simulink model "ACDCMG_woPV"  (R2022a)
settings: Solver=FixedStepAuto  StartTime=0.0  StopTime=0.2  FixedStep=Ts  MaxStep=1e-2  RelTol=1e-3
InitFcn:
  | Set_parameters_R2018
values from neighbouring files (symbols this model uses):
  D_invs = 0.05    [Set_parameters_R2018.m]
  dis11 = 3    [Set_parameters_R2018.m]
  dis14 = 2    [Set_parameters_R2018.m]
  dis2 = 0.2    [Set_parameters_R2018.m]
  dis3 = 0.15    [Set_parameters_R2018.m]
  dis4 = 0.4    [Set_parameters_R2018.m]
  dis5 = 0.4    [Set_parameters_R2018.m]
  dis6 = 0.4    [Set_parameters_R2018.m]
  dis8 = 2    [Set_parameters_R2018.m]
  Fnom = 60    [Set_parameters_R2018.m]
  H_invs = 6    [Set_parameters_R2018.m]
  max_min = 1    [Set_parameters_R2018.m]
  P_Load_3 = S_Load_3* PF_Load_3    (= 25500)    [Set_parameters_R2018.m]
  P_nom_inv = 3e3    (= 3000)    [Set_parameters_R2018.m]
  Pnom_T1 = 1.5e6    (= 1500000)    [Set_parameters_R2018.m]
  Pnom_T2 = 1.5e6    (= 1500000)    [Set_parameters_R2018.m]
  Pnom_T3 = 4e6    (= 4000000)    [Set_parameters_R2018.m]
  Ql_Load_3 = S_Load_3 * sin(acos(PF_Load_3))    [Set_parameters_R2018.m]
  R_Load_9 = (Vnom_prim * 1.35)^2 / P_Load_9    (= 1084.6153125)    [Set_parameters_R2018.m]
  R_Load_DC = Vnom_DC^2/ P_Load_DC    (= 45)    [Set_parameters_R2018.m]
  Rl = 0.394    [Set_parameters_R2018.m]
  Rls = 0.198    [Set_parameters_R2018.m]
  Ts = Ts_Power    (= 6.94444444444e-06)    [Set_parameters_R2018.m]
  Ts_Control = 6*Ts_Power    (= 4.16666666667e-05)    [Set_parameters_R2018.m]
  Ts_Power = 1/(24*Fnom)/100    (= 6.94444444444e-06)    [Set_parameters_R2018.m]
  V1_LL_T3 = 69e3    (= 69000)    [Set_parameters_R2018.m]
  Vnom_DC = 300    [Set_parameters_R2018.m]
  Vnom_Diesel = 2.4e3    (= 2400)    [Set_parameters_R2018.m]
  Vnom_prim = 13.8e3    (= 13800)    [Set_parameters_R2018.m]
  Vnom_sec = 220    [Set_parameters_R2018.m]
  Vnom_ter_AC_DC = 150    [Set_parameters_R2018.m]
  Xl = 0.1168    [Set_parameters_R2018.m]
  Xls = 0.1089    [Set_parameters_R2018.m]
undefined symbols (not defined in the file or in its folder): D1, Delta, DiscIntNeverNeededParam, ee_sli_rtmsupport, fn, gcbh, Ion, Lithium, S, sigbuilder_block, VnInv
libraries: powerlib_extras x55, spsCurrentMeasurementLib x53, powerlib_meascontrol x42, spsSeriesRLCBranchLib x32, spsVoltageMeasurementLib x31, spsRMSLib x29, spsThreePhaseVIMeasurementLib x24, simulink x21, spsThreePhaseSeriesRLCBranchLib x19, spsPower3phInstantaneousLib x15, spsPowerLib x12, spsGroundLib x11
(part 5 of 9)

== system ACDCMG_woPV/Grid Bi-directional Converter 1.1 300 (DC) // 150 V (AC) P_nom 3kW/Control of Inverter ==
  note: VL-L rms_1
  note: Primary control
  note: Control of Inverter
  Means : Inport
  Bus Selector : BusSelector  OutputSignals=signal1,signal2,signal3,signal4
  Discrete PWM Generator1 : Subsystem  AncestorBlock=|  DialogController=POWERSYS.PowerSysDialog  mask(Discrete PWM Generator){GeneratorMode=3-arm  bridge (6 pulses), Fc=4000, Ts=Ts_Power, Internal=off, mIndex=0.99, Freq=60, Phase=0}
      | powerlib_extras/Discrete 
      | Control Blocks/Discrete
      | PWM Generator
      mask prompts: GeneratorMode "Generator Mode"; Fc "Carrier frequency (Hz):"; Ts "Sample time:"; Internal "Internal generation of modulating signal(s)"; mIndex "Modulation index  (0<m<1) :"; Freq "Frequency of output voltage (Hz)"; Phase "Phase of output voltage (degrees)"
      mask help:
      | This discrete block generates pulses for carrier-based PWM (Pulse Width Modulation), self-commutated IGBTs,GTOs or FETs bridges.
      |
      | Depending on the number of bridge arms selected in the "Generator Mode" parameter, the block can be used either for single-phase or three-phase PWM control.
      mask init:
      | powericon('psbcallbacks',gcb,'Discrete PWM Generator');
      | if Freq==0
      |     Phase=90;
      | end
      | switch GeneratorMode
      | case 1,
      |     Internal_Phase=0;
      |    Signal_PortWidth=1;
      |    Select1_Elements=[1 2];
      |    Select1_PortWidth=2;
      |    Select3_Elements=[1 2];
      |    Select3_PortWidth=4;
      | case 2,
      |     Internal_Phase=0;
      |     Signal_PortWidth=1;
      |     Select1_Elements=[1 2];
      |     Select1_PortWidth=2;
      |     Select3_Elements=[1 2 3 4];
      |     Select3_PortWidth=4;
      | case 3,
      |     Internal_Phase=[0 -2*pi/3 2*pi/3];
      |     Signal_PortWidth=3;
      |     Select1_Elements=[1 4 2 5 3 6];
      |     Select1_PortWidth=6;
      |    Select3_Elements=[1 2 3 4 5 6];
      |    Select3_PortWidth=12;
      | case 4,
      |     Internal_Phase=[0 -2*pi/3 2*pi/3];
      |     Signal_PortWidth=3;
      |     Select1_Elements=[1 4 2 5 3 6];
      |     Select1_PortWidth=6;
      |    Select3_Elements=[1 2 3 4 5 6 7 8 9 10 11 12];
      |    Select3_PortWidth=12;
      | end
      | power_initmask();
      mask Help:
      | The output pulses are a vector (with values=0 or 1). Depending on the selected "Generator Mode", the output vector contains:
      | For a 1-arm  bridge: Two pulses. Pulse 1 is for the upper switch and pulse 2 is for the lower switch.
      | For a 2-arm  bridge: Four pulses. Pulses 1 and 3 are respectively for the upper switches of the first and second arm. Pulses 2 and 4 are for the lower switches.
      | For a 3-arm  bridge: Six pulses. Pulses 1,3 and 5 are respectively for the upper switches of the first,second and third arm. Pulses 2,4 and 6 are for the lower switches.
      | For double 3-arm bridges: Twelve pulses.The first six pulses (pulses 1 to 6) must be sent to the first 3-arm bridge and the last six (pulses 7 to 12) to the second 3-arm bridge.
      | 
      | By selecting "Internal generation" you can can control the modulation index m, frequency and phase of the output voltage  from the internal parameters (m, Freq and Phase). Otherwise, external signals are used for pulse generation. The width of the input vector must be 1 for single phase bridges ( 1-arm or 2-arm)  and 3 for 3-phase bridges  (single or double bridge).
      mask TypeOptions GeneratorMode: 1-arm  bridge (2 pulses) | 2-arm  bridge (4 pulses) | 3-arm  bridge (6 pulses) | Double 3-arm  bridges (12 pulses)
      mask Callback Internal: powericon('psbcallbacks',gcb,'Discrete PWM Generator',[]);
  MI Controller : Subsystem
  Unit Delay4 : UnitDelay  SampleTime=Ts_Power  HasFrameUpgradeWarning=on
  VL-L_1 : Scope  NumInputPorts=2
  Vph_abc : Scope
  Vph_rms_1 : Scope
  u / m : Scope
  Pulses : Outport  VectorParamsAs1DForOutWhenUnconnected=off
  wires:
  MI Controller/2(u / m) -> u / m/1
  Unit Delay4/1 -> Pulses/1
  Discrete PWM Generator1/1(Pulses) -> Unit Delay4/1
  Bus Selector/1 -> Vph_abc/1, MI Controller/1(Vabc)  "<signal1>"
  Bus Selector/2 -> VL-L_1/1  "<signal2>"
  Bus Selector/3 -> VL-L_1/2  "<signal3>"
  Bus Selector/4 -> Vph_rms_1/1  "<signal4>"
  Means/1 -> Bus Selector/1
  MI Controller/1(Vabc_inv) -> Discrete PWM Generator1/1(Uref)

== system ACDCMG_woPV/Grid Bi-directional Converter 1.1 300 (DC) // 150 V (AC) P_nom 3kW1/Control of Inverter ==
  note: VL-L rms_1
  note: Primary control
  note: Control of Inverter
  Means : Inport
  Bus Selector : BusSelector  OutputSignals=signal1,signal2,signal3,signal4
  Discrete PWM Generator1 : Subsystem  AncestorBlock=|  DialogController=POWERSYS.PowerSysDialog  mask(Discrete PWM Generator){GeneratorMode=3-arm  bridge (6 pulses), Fc=4000, Ts=Ts_Power, Internal=off, mIndex=0.99, Freq=60, Phase=0}
      | powerlib_extras/Discrete 
      | Control Blocks/Discrete
      | PWM Generator
      mask prompts: GeneratorMode "Generator Mode"; Fc "Carrier frequency (Hz):"; Ts "Sample time:"; Internal "Internal generation of modulating signal(s)"; mIndex "Modulation index  (0<m<1) :"; Freq "Frequency of output voltage (Hz)"; Phase "Phase of output voltage (degrees)"
      mask help:
      | This discrete block generates pulses for carrier-based PWM (Pulse Width Modulation), self-commutated IGBTs,GTOs or FETs bridges.
      |
      | Depending on the number of bridge arms selected in the "Generator Mode" parameter, the block can be used either for single-phase or three-phase PWM control.
      mask init: same as ACDCMG_woPV/Grid Bi-directional Converter 1.1 300 (DC) // 150 V (AC) P_nom 3kW/Control of Inverter/Discrete PWM Generator1
      mask Help:
      | The output pulses are a vector (with values=0 or 1). Depending on the selected "Generator Mode", the output vector contains:
      | For a 1-arm  bridge: Two pulses. Pulse 1 is for the upper switch and pulse 2 is for the lower switch.
      | For a 2-arm  bridge: Four pulses. Pulses 1 and 3 are respectively for the upper switches of the first and second arm. Pulses 2 and 4 are for the lower switches.
      | For a 3-arm  bridge: Six pulses. Pulses 1,3 and 5 are respectively for the upper switches of the first,second and third arm. Pulses 2,4 and 6 are for the lower switches.
      | For double 3-arm bridges: Twelve pulses.The first six pulses (pulses 1 to 6) must be sent to the first 3-arm bridge and the last six (pulses 7 to 12) to the second 3-arm bridge.
      | 
      | By selecting "Internal generation" you can can control the modulation index m, frequency and phase of the output voltage  from the internal parameters (m, Freq and Phase). Otherwise, external signals are used for pulse generation. The width of the input vector must be 1 for single phase bridges ( 1-arm or 2-arm)  and 3 for 3-phase bridges  (single or double bridge).
      mask TypeOptions GeneratorMode: 1-arm  bridge (2 pulses) | 2-arm  bridge (4 pulses) | 3-arm  bridge (6 pulses) | Double 3-arm  bridges (12 pulses)
      mask Callback Internal: powericon('psbcallbacks',gcb,'Discrete PWM Generator',[]);
  MI Controller : Subsystem
  Unit Delay4 : UnitDelay  SampleTime=Ts_Power  HasFrameUpgradeWarning=on
  VL-L_1 : Scope  NumInputPorts=2
  Vph_abc : Scope
  Vph_rms_1 : Scope
  u / m : Scope
  Pulses : Outport  VectorParamsAs1DForOutWhenUnconnected=off
  wires:
  MI Controller/2(u / m) -> u / m/1
  Unit Delay4/1 -> Pulses/1
  Discrete PWM Generator1/1(Pulses) -> Unit Delay4/1
  Bus Selector/1 -> Vph_abc/1, MI Controller/1(Vabc)  "<signal1>"
  Bus Selector/2 -> VL-L_1/1  "<signal2>"
  Bus Selector/3 -> VL-L_1/2  "<signal3>"
  Bus Selector/4 -> Vph_rms_1/1  "<signal4>"
  Means/1 -> Bus Selector/1
  MI Controller/1(Vabc_inv) -> Discrete PWM Generator1/1(Uref)

== system ACDCMG_woPV/Grid Bi-directional Converter 1.1 300 (DC) // 150 V (AC) P_nom 3kW2/Control of Inverter ==
  note: VL-L rms_1
  note: Primary control
  note: Control of Inverter
  Means : Inport
  Bus Selector : BusSelector  OutputSignals=signal1,signal2,signal3,signal4
  Discrete PWM Generator1 : Subsystem  AncestorBlock=|  DialogController=POWERSYS.PowerSysDialog  mask(Discrete PWM Generator){GeneratorMode=3-arm  bridge (6 pulses), Fc=4000, Ts=Ts_Power, Internal=off, mIndex=0.99, Freq=60, Phase=0}
      | powerlib_extras/Discrete 
      | Control Blocks/Discrete
      | PWM Generator
      mask prompts: GeneratorMode "Generator Mode"; Fc "Carrier frequency (Hz):"; Ts "Sample time:"; Internal "Internal generation of modulating signal(s)"; mIndex "Modulation index  (0<m<1) :"; Freq "Frequency of output voltage (Hz)"; Phase "Phase of output voltage (degrees)"
      mask help:
      | This discrete block generates pulses for carrier-based PWM (Pulse Width Modulation), self-commutated IGBTs,GTOs or FETs bridges.
      |
      | Depending on the number of bridge arms selected in the "Generator Mode" parameter, the block can be used either for single-phase or three-phase PWM control.
      mask init: same as ACDCMG_woPV/Grid Bi-directional Converter 1.1 300 (DC) // 150 V (AC) P_nom 3kW/Control of Inverter/Discrete PWM Generator1
      mask Help:
      | The output pulses are a vector (with values=0 or 1). Depending on the selected "Generator Mode", the output vector contains:
      | For a 1-arm  bridge: Two pulses. Pulse 1 is for the upper switch and pulse 2 is for the lower switch.
      | For a 2-arm  bridge: Four pulses. Pulses 1 and 3 are respectively for the upper switches of the first and second arm. Pulses 2 and 4 are for the lower switches.
      | For a 3-arm  bridge: Six pulses. Pulses 1,3 and 5 are respectively for the upper switches of the first,second and third arm. Pulses 2,4 and 6 are for the lower switches.
      | For double 3-arm bridges: Twelve pulses.The first six pulses (pulses 1 to 6) must be sent to the first 3-arm bridge and the last six (pulses 7 to 12) to the second 3-arm bridge.
      | 
      | By selecting "Internal generation" you can can control the modulation index m, frequency and phase of the output voltage  from the internal parameters (m, Freq and Phase). Otherwise, external signals are used for pulse generation. The width of the input vector must be 1 for single phase bridges ( 1-arm or 2-arm)  and 3 for 3-phase bridges  (single or double bridge).
      mask TypeOptions GeneratorMode: 1-arm  bridge (2 pulses) | 2-arm  bridge (4 pulses) | 3-arm  bridge (6 pulses) | Double 3-arm  bridges (12 pulses)
      mask Callback Internal: powericon('psbcallbacks',gcb,'Discrete PWM Generator',[]);
  MI Controller : Subsystem
  Unit Delay4 : UnitDelay  SampleTime=Ts_Power  HasFrameUpgradeWarning=on
  VL-L_1 : Scope  NumInputPorts=2
  Vph_abc : Scope
  Vph_rms_1 : Scope
  u / m : Scope
  Pulses : Outport  VectorParamsAs1DForOutWhenUnconnected=off
  wires:
  MI Controller/2(u / m) -> u / m/1
  Unit Delay4/1 -> Pulses/1
  Discrete PWM Generator1/1(Pulses) -> Unit Delay4/1
  Bus Selector/1 -> Vph_abc/1, MI Controller/1(Vabc)  "<signal1>"
  Bus Selector/2 -> VL-L_1/1  "<signal2>"
  Bus Selector/3 -> VL-L_1/2  "<signal3>"
  Bus Selector/4 -> Vph_rms_1/1  "<signal4>"
  Means/1 -> Bus Selector/1
  MI Controller/1(Vabc_inv) -> Discrete PWM Generator1/1(Uref)

== system ACDCMG_woPV/Grid Bi-directional Converter 1.2 300 (DC) // 150 V (AC) P_nom 3kW/Control of Inverter ==
  note: VL-L rms_2
  note: Primary control
  note: Control of Inverter
  Bus Selector : BusSelector  Commented=on  OutputSignals=signal1,signal2,signal3,signal4
  Demux3 : Demux  Outputs=3
  Demux4 : Demux  Outputs=3
  Discrete PWM Generator1 : Subsystem  Commented=on  AncestorBlock=|  DialogController=POWERSYS.PowerSysDialog  mask(Discrete PWM Generator){GeneratorMode=3-arm  bridge (6 pulses), Fc=4000, Ts=Ts_Power, Internal=off, mIndex=0.99, Freq=60, Phase=0}
      | powerlib_extras/Discrete 
      | Control Blocks/Discrete
      | PWM Generator
      mask prompts: GeneratorMode "Generator Mode"; Fc "Carrier frequency (Hz):"; Ts "Sample time:"; Internal "Internal generation of modulating signal(s)"; mIndex "Modulation index  (0<m<1) :"; Freq "Frequency of output voltage (Hz)"; Phase "Phase of output voltage (degrees)"
      mask help:
      | This discrete block generates pulses for carrier-based PWM (Pulse Width Modulation), self-commutated IGBTs,GTOs or FETs bridges.
      |
      | Depending on the number of bridge arms selected in the "Generator Mode" parameter, the block can be used either for single-phase or three-phase PWM control.
      mask init: same as ACDCMG_woPV/Grid Bi-directional Converter 1.1 300 (DC) // 150 V (AC) P_nom 3kW/Control of Inverter/Discrete PWM Generator1
      mask Help:
      | The output pulses are a vector (with values=0 or 1). Depending on the selected "Generator Mode", the output vector contains:
      | For a 1-arm  bridge: Two pulses. Pulse 1 is for the upper switch and pulse 2 is for the lower switch.
      | For a 2-arm  bridge: Four pulses. Pulses 1 and 3 are respectively for the upper switches of the first and second arm. Pulses 2 and 4 are for the lower switches.
      | For a 3-arm  bridge: Six pulses. Pulses 1,3 and 5 are respectively for the upper switches of the first,second and third arm. Pulses 2,4 and 6 are for the lower switches.
      | For double 3-arm bridges: Twelve pulses.The first six pulses (pulses 1 to 6) must be sent to the first 3-arm bridge and the last six (pulses 7 to 12) to the second 3-arm bridge.
      | 
      | By selecting "Internal generation" you can can control the modulation index m, frequency and phase of the output voltage  from the internal parameters (m, Freq and Phase). Otherwise, external signals are used for pulse generation. The width of the input vector must be 1 for single phase bridges ( 1-arm or 2-arm)  and 3 for 3-phase bridges  (single or double bridge).
      mask TypeOptions GeneratorMode: 1-arm  bridge (2 pulses) | 2-arm  bridge (4 pulses) | 3-arm  bridge (6 pulses) | Double 3-arm  bridges (12 pulses)
      mask Callback Internal: powericon('psbcallbacks',gcb,'Discrete PWM Generator',[]);
  Goto : Goto  Commented=on  GotoTag=PWM
  MI Controller : Subsystem  Commented=on
  Mux2 : Mux  Inputs=2
  PQ_B1 : Scope
  "P_Q(kW, kvar)1" : Display
      settings: Format=bank  Decimation=2000
  Positive-Sequence Active & Reactive Power1 : Subsystem  AncestorBlock=|  DialogController=POWERSYS.PowerSysDialog  mask(Discrete 3-phase Positive-Sequence Active & Reactive Power){Freq=60, Par_Vinit=[0 0], Par_Iinit=[0 0], Ts=5e-6}
      | powerlib_extras/Discrete
      | Measurements/Discrete 3-phase 
      | Positive-Sequence 
      | Active & Reactive Power
      mask prompts: Freq "Fundamental frequency (Hz):"; Par_Vinit "Voltage initial input: [ Mag  Phase(degrees) ]"; Par_Iinit "Current initial input: [ Mag  Phase(degrees) ]"; Ts "Sample time:"
      mask help:
      | Measure the three-phase active power P and reactive power Q associated with a periodic set of three-phase voltages and currents which may contain harmonics. P and Q are calculated by evaluating the fundamental values (positive-sequence) of the input voltages and currents with a running window over one cycle of the fundamental frequency.
      |
      | Current flowing into an RL circuit will produce  positive active and reactive powers.
      |
      | Vabc input: Three-phase instantaneous voltage (V)
      | Iabc input: Three-phase instantaneous current (A)
      |
      | Output 1: Vector [Mag_V(V) Mag_I(A)] of the fundamental values of the voltage & current (peak values of the positive-sequence)
      | Output 2: 3-phase PQ measurement vector [P(W) Q (var)] evaluated at the fundamental frequency.
      |
      | For the first cycle of simulation, the outputs are held constant using the values specified by the parameters "Initial input".
      mask init:
      | power_initmask();
      mask Help: This block is part of a subset of blocks in the Extras library that does not have documentation associated with it, other than the block mask description.
      mask Display: disp('')
  RMS_VI2 : Scope
  RMS_V_I1 : Display
      settings: Format=bank  Decimation=2000
  Scope1 : Scope  NumInputPorts=2
  Scope2 : Scope
  Scope6 : Scope  NumInputPorts=2
  Terminator{1..6} (6 alike) : Terminator
  Unit Delay4 : UnitDelay  Commented=on  SampleTime=Ts_Power  HasFrameUpgradeWarning=on
  V/F : Subsystem
  VL-L_2 : Scope  Commented=on  NumInputPorts=2
  Vph_rms_2 : Scope  Commented=on
  m2 : Scope  Commented=on
  m_2 : Scope  Commented=on
  Pulses : Outport  VectorParamsAs1DForOutWhenUnconnected=off
  wires:
  MI Controller/2(m) -> m_2/1
  Discrete PWM Generator1/1(Pulses) -> Unit Delay4/1
  MI Controller/1(Vabc_inv) -> Discrete PWM Generator1/1(Uref)
  Bus Selector/1 -> m2/1, MI Controller/1(Vabc)  "<signal1>"
  Bus Selector/2 -> VL-L_2/1  "<signal2>"
  Bus Selector/3 -> VL-L_2/2  "<signal3>"
  Bus Selector/4 -> Vph_rms_2/1  "<signal4>"
  [Udc] -> V/F/4(Udc)
  Demux3/2 -> Terminator1/1
  Demux4/3 -> Terminator6/1
  [i] -> V/F/3(i)
  Demux4/2 -> Terminator5/1
  Demux4/1 -> Mux2/2
  Demux3/3 -> Terminator4/1
  [io] -> Scope1/2, Positive-Sequence Active & Reactive Power1/2(Iabc)
  Mux2/1 -> Scope2/1
  Demux3/1 -> Mux2/1
  Positive-Sequence Active & Reactive Power1/2(P_Q(kW)) -> PQ_B1/1, "P_Q(kW, kvar)1"/1
  Positive-Sequence Active & Reactive Power1/4(PF) -> Terminator3/1
  Positive-Sequence Active & Reactive Power1/3(Phase_V_I) -> Terminator2/1
  Positive-Sequence Active & Reactive Power1/1(RMS_V_I) -> RMS_V_I1/1, RMS_VI2/1
  [e] -> Scope1/1, Positive-Sequence Active & Reactive Power1/1(Vabc)
  [e] -> Scope6/1, Demux3/1, V/F/1(e)
  [io] -> Scope6/2, Demux4/1, V/F/2(io)
  V/F/1(Pulses) -> Pulses/1

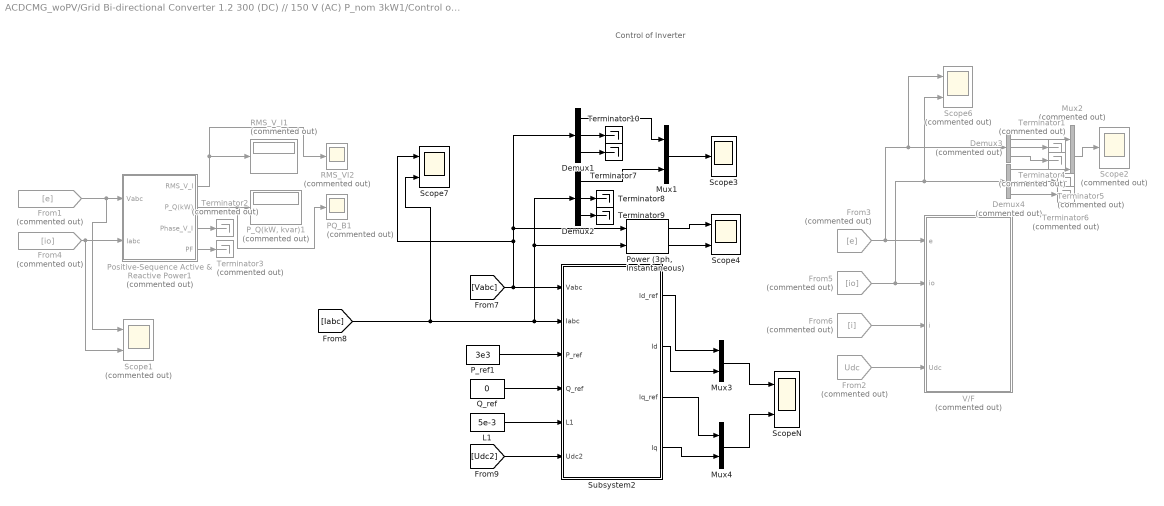
== system ACDCMG_woPV/Grid Bi-directional Converter 1.2 300 (DC) // 150 V (AC) P_nom 3kW1/Control of Inverter ==
  note: Control of Inverter
  Demux1 : Demux  Outputs=3
  Demux2 : Demux  Outputs=3
  Demux3 : Demux  Commented=on  Outputs=3
  Demux4 : Demux  Commented=on  Outputs=3
  From1 : From  Commented=on  GotoTag=e  TagVisibility=global
      settings: CloseFcn=tagdialog Close
  From2 : From  Commented=on  GotoTag=Udc  TagVisibility=global
  From3 : From  Commented=on  GotoTag=e  TagVisibility=global
  From4 : From  Commented=on  GotoTag=io  TagVisibility=global
      settings: CloseFcn=tagdialog Close
  From5 : From  Commented=on  GotoTag=io  TagVisibility=global
  From6 : From  Commented=on  GotoTag=i  TagVisibility=global
  L1 : Constant  Value=5e-3
  Mux1 : Mux  Inputs=2
  Mux2 : Mux  Commented=on  Inputs=2
  Mux3 : Mux  Inputs=2
  Mux4 : Mux  Inputs=2
  PQ_B1 : Scope  Commented=on
  "P_Q(kW, kvar)1" : Display  Commented=on
      settings: Format=bank  Decimation=2000
  P_ref1 : Constant  Value=3e3
  Positive-Sequence Active & Reactive Power1 : Subsystem  Commented=on  AncestorBlock=|  DialogController=POWERSYS.PowerSysDialog  mask(Discrete 3-phase Positive-Sequence Active & Reactive Power){Freq=60, Par_Vinit=[0 0], Par_Iinit=[0 0], Ts=5e-6}
      | powerlib_extras/Discrete
      | Measurements/Discrete 3-phase 
      | Positive-Sequence 
      | Active & Reactive Power
      mask prompts: Freq "Fundamental frequency (Hz):"; Par_Vinit "Voltage initial input: [ Mag  Phase(degrees) ]"; Par_Iinit "Current initial input: [ Mag  Phase(degrees) ]"; Ts "Sample time:"
      mask help:
      | Measure the three-phase active power P and reactive power Q associated with a periodic set of three-phase voltages and currents which may contain harmonics. P and Q are calculated by evaluating the fundamental values (positive-sequence) of the input voltages and currents with a running window over one cycle of the fundamental frequency.
      |
      | Current flowing into an RL circuit will produce  positive active and reactive powers.
      |
      | Vabc input: Three-phase instantaneous voltage (V)
      | Iabc input: Three-phase instantaneous current (A)
      |
      | Output 1: Vector [Mag_V(V) Mag_I(A)] of the fundamental values of the voltage & current (peak values of the positive-sequence)
      | Output 2: 3-phase PQ measurement vector [P(W) Q (var)] evaluated at the fundamental frequency.
      |
      | For the first cycle of simulation, the outputs are held constant using the values specified by the parameters "Initial input".
      mask init:
      | power_initmask();
      mask Help: This block is part of a subset of blocks in the Extras library that does not have documentation associated with it, other than the block mask description.
      mask Display: disp('')
  "Power (3ph, Instantaneous)" : powerlib_meascontrol/Measurements/Power (3ph, Instantaneous)
  Q_ref : Constant  Value=0
  RMS_VI2 : Scope  Commented=on
  RMS_V_I1 : Display  Commented=on
      settings: Format=bank  Decimation=2000
  Scope1 : Scope  Commented=on  NumInputPorts=2
  Scope2 : Scope  Commented=on
  Scope3 : Scope
  Scope4 : Scope  NumInputPorts=2
  Scope6 : Scope  Commented=on  NumInputPorts=2
  Scope7 : Scope  NumInputPorts=2
  ScopeN : Scope  NumInputPorts=2
  Subsystem2 : Subsystem  mask{Kp=21, Ki=101, Kd=0}
      mask prompts: Kp "Proportional gain (Kp):"; Ki "Integral gain (Ki):"; Kd "Derivative gain (Kd):"
  Terminator{1..6} (6 alike) : Terminator  Commented=on
  Terminator{7..10} (4 alike) : Terminator
  V/F : Subsystem  Commented=on
  wires:
  From2/1 -> V/F/4(Udc)
  Demux3/2 -> Terminator1/1
  Demux4/3 -> Terminator6/1
  From6/1 -> V/F/3(i)
  Demux4/2 -> Terminator5/1
  Demux4/1 -> Mux2/2
  Demux3/3 -> Terminator4/1
  From4/1 -> Scope1/2, Positive-Sequence Active & Reactive Power1/2(Iabc)
  Mux2/1 -> Scope2/1
  Demux3/1 -> Mux2/1
  Positive-Sequence Active & Reactive Power1/2(P_Q(kW)) -> PQ_B1/1, "P_Q(kW, kvar)1"/1
  Positive-Sequence Active & Reactive Power1/4(PF) -> Terminator3/1
  Positive-Sequence Active & Reactive Power1/3(Phase_V_I) -> Terminator2/1
  Positive-Sequence Active & Reactive Power1/1(RMS_V_I) -> RMS_V_I1/1, RMS_VI2/1
  From1/1 -> Scope1/1, Positive-Sequence Active & Reactive Power1/1(Vabc)
  From3/1 -> Scope6/1, Demux3/1, V/F/1(e)
  From5/1 -> Scope6/2, Demux4/1, V/F/2(io)
  Q_ref/1 -> Subsystem2/4(Q_ref)
  [Vabc] -> Subsystem2/1(Vabc), Scope7/1, Demux1/1, "Power (3ph, Instantaneous)"/1
  Demux2/3 -> Terminator9/1
  Demux1/2 -> Terminator10/1
  [Udc2] -> Subsystem2/6(Udc2)
  P_ref1/1 -> Subsystem2/3(P_ref)
  Demux2/2 -> Terminator8/1
  "Power (3ph, Instantaneous)"/2 -> Scope4/2
  "Power (3ph, Instantaneous)"/1 -> Scope4/1
  Subsystem2/3(Iq_ref) -> Mux4/1
  Subsystem2/2(Id) -> Mux3/2
  Demux2/1 -> Mux1/2
  Mux1/1 -> Scope3/1
  L1/1 -> Subsystem2/5(L1)
  Mux3/1 -> ScopeN/1
  Subsystem2/4(Iq) -> Mux4/2
  [Iabc] -> Scope7/2, Demux2/1, "Power (3ph, Instantaneous)"/2, Subsystem2/2(Iabc)
  Subsystem2/1(Id_ref) -> Mux3/1
  Mux4/1 -> ScopeN/2
  Demux1/3 -> Terminator7/1
  Demux1/1 -> Mux1/1

== system ACDCMG_woPV/Grid Bi-directional Converter 1.2 300 (DC) // 150 V (AC) P_nom 3kW1/Power Measurement (Three-Phase) ==
  V : Inport
  I : Inport  Port=2
  Continuous : Subsystem  VariantControl=Continuous
  Discrete : Subsystem  VariantControl=Discrete
  P : Outport  VectorParamsAs1DForOutWhenUnconnected=off
  Q : Outport  Port=2  VectorParamsAs1DForOutWhenUnconnected=off

== system ACDCMG_woPV/Grid Bi-directional Converter 1.2 300 (DC) // 150 V (AC) P_nom 3kW2/Control of Inverter ==
  note: VL-L rms_2
  note: Primary control
  note: Control of Inverter
  Bus Selector : BusSelector  Commented=on  OutputSignals=signal1,signal2,signal3,signal4
  Demux3 : Demux  Outputs=3
  Demux4 : Demux  Outputs=3
  Discrete PWM Generator1 : Subsystem  Commented=on  AncestorBlock=|  DialogController=POWERSYS.PowerSysDialog  mask(Discrete PWM Generator){GeneratorMode=3-arm  bridge (6 pulses), Fc=4000, Ts=Ts_Power, Internal=off, mIndex=0.99, Freq=60, Phase=0}
      | powerlib_extras/Discrete 
      | Control Blocks/Discrete
      | PWM Generator
      mask prompts: GeneratorMode "Generator Mode"; Fc "Carrier frequency (Hz):"; Ts "Sample time:"; Internal "Internal generation of modulating signal(s)"; mIndex "Modulation index  (0<m<1) :"; Freq "Frequency of output voltage (Hz)"; Phase "Phase of output voltage (degrees)"
      mask help:
      | This discrete block generates pulses for carrier-based PWM (Pulse Width Modulation), self-commutated IGBTs,GTOs or FETs bridges.
      |
      | Depending on the number of bridge arms selected in the "Generator Mode" parameter, the block can be used either for single-phase or three-phase PWM control.
      mask init: same as ACDCMG_woPV/Grid Bi-directional Converter 1.1 300 (DC) // 150 V (AC) P_nom 3kW/Control of Inverter/Discrete PWM Generator1
      mask Help:
      | The output pulses are a vector (with values=0 or 1). Depending on the selected "Generator Mode", the output vector contains:
      | For a 1-arm  bridge: Two pulses. Pulse 1 is for the upper switch and pulse 2 is for the lower switch.
      | For a 2-arm  bridge: Four pulses. Pulses 1 and 3 are respectively for the upper switches of the first and second arm. Pulses 2 and 4 are for the lower switches.
      | For a 3-arm  bridge: Six pulses. Pulses 1,3 and 5 are respectively for the upper switches of the first,second and third arm. Pulses 2,4 and 6 are for the lower switches.
      | For double 3-arm bridges: Twelve pulses.The first six pulses (pulses 1 to 6) must be sent to the first 3-arm bridge and the last six (pulses 7 to 12) to the second 3-arm bridge.
      | 
      | By selecting "Internal generation" you can can control the modulation index m, frequency and phase of the output voltage  from the internal parameters (m, Freq and Phase). Otherwise, external signals are used for pulse generation. The width of the input vector must be 1 for single phase bridges ( 1-arm or 2-arm)  and 3 for 3-phase bridges  (single or double bridge).
      mask TypeOptions GeneratorMode: 1-arm  bridge (2 pulses) | 2-arm  bridge (4 pulses) | 3-arm  bridge (6 pulses) | Double 3-arm  bridges (12 pulses)
      mask Callback Internal: powericon('psbcallbacks',gcb,'Discrete PWM Generator',[]);
  Goto : Goto  Commented=on  GotoTag=PWM
  MI Controller : Subsystem  Commented=on
  Mux2 : Mux  Inputs=2
  PQ_B1 : Scope
  "P_Q(kW, kvar)1" : Display
      settings: Format=bank  Decimation=2000
  Positive-Sequence Active & Reactive Power1 : Subsystem  AncestorBlock=|  DialogController=POWERSYS.PowerSysDialog  mask(Discrete 3-phase Positive-Sequence Active & Reactive Power){Freq=60, Par_Vinit=[0 0], Par_Iinit=[0 0], Ts=5e-6}
      | powerlib_extras/Discrete
      | Measurements/Discrete 3-phase 
      | Positive-Sequence 
      | Active & Reactive Power
      mask prompts: Freq "Fundamental frequency (Hz):"; Par_Vinit "Voltage initial input: [ Mag  Phase(degrees) ]"; Par_Iinit "Current initial input: [ Mag  Phase(degrees) ]"; Ts "Sample time:"
      mask help:
      | Measure the three-phase active power P and reactive power Q associated with a periodic set of three-phase voltages and currents which may contain harmonics. P and Q are calculated by evaluating the fundamental values (positive-sequence) of the input voltages and currents with a running window over one cycle of the fundamental frequency.
      |
      | Current flowing into an RL circuit will produce  positive active and reactive powers.
      |
      | Vabc input: Three-phase instantaneous voltage (V)
      | Iabc input: Three-phase instantaneous current (A)
      |
      | Output 1: Vector [Mag_V(V) Mag_I(A)] of the fundamental values of the voltage & current (peak values of the positive-sequence)
      | Output 2: 3-phase PQ measurement vector [P(W) Q (var)] evaluated at the fundamental frequency.
      |
      | For the first cycle of simulation, the outputs are held constant using the values specified by the parameters "Initial input".
      mask init:
      | power_initmask();
      mask Help: This block is part of a subset of blocks in the Extras library that does not have documentation associated with it, other than the block mask description.
      mask Display: disp('')
  RMS_VI2 : Scope
  RMS_V_I1 : Display
      settings: Format=bank  Decimation=2000
  Scope1 : Scope  NumInputPorts=2
  Scope2 : Scope
  Scope6 : Scope  NumInputPorts=2
  Terminator{1..6} (6 alike) : Terminator
  Unit Delay4 : UnitDelay  Commented=on  SampleTime=Ts_Power  HasFrameUpgradeWarning=on
  V/F : Subsystem
  VL-L_2 : Scope  Commented=on  NumInputPorts=2
  Vph_rms_2 : Scope  Commented=on
  m2 : Scope  Commented=on
  m_2 : Scope  Commented=on
  Pulses : Outport  VectorParamsAs1DForOutWhenUnconnected=off
  wires:
  MI Controller/2(m) -> m_2/1
  Discrete PWM Generator1/1(Pulses) -> Unit Delay4/1
  MI Controller/1(Vabc_inv) -> Discrete PWM Generator1/1(Uref)
  Bus Selector/1 -> m2/1, MI Controller/1(Vabc)  "<signal1>"
  Bus Selector/2 -> VL-L_2/1  "<signal2>"
  Bus Selector/3 -> VL-L_2/2  "<signal3>"
  Bus Selector/4 -> Vph_rms_2/1  "<signal4>"
  [Udc] -> V/F/4(Udc)
  Demux3/2 -> Terminator1/1
  Demux4/3 -> Terminator6/1
  [i] -> V/F/3(i)
  Demux4/2 -> Terminator5/1
  Demux4/1 -> Mux2/2
  Demux3/3 -> Terminator4/1
  [io] -> Scope1/2, Positive-Sequence Active & Reactive Power1/2(Iabc)
  Mux2/1 -> Scope2/1
  Demux3/1 -> Mux2/1
  Positive-Sequence Active & Reactive Power1/2(P_Q(kW)) -> PQ_B1/1, "P_Q(kW, kvar)1"/1
  Positive-Sequence Active & Reactive Power1/4(PF) -> Terminator3/1
  Positive-Sequence Active & Reactive Power1/3(Phase_V_I) -> Terminator2/1
  Positive-Sequence Active & Reactive Power1/1(RMS_V_I) -> RMS_V_I1/1, RMS_VI2/1
  [e] -> Scope1/1, Positive-Sequence Active & Reactive Power1/1(Vabc)
  [e] -> Scope6/1, Demux3/1, V/F/1(e)
  [io] -> Scope6/2, Demux4/1, V/F/2(io)
  V/F/1(Pulses) -> Pulses/1

== system ACDCMG_woPV/Grid Bi-directional Converter 1.2 300 (DC) // 150 V (AC) P_nom 3kW3/Control of Inverter ==
  note: Control of Inverter
  Demux3 : Demux  Outputs=3
  Demux4 : Demux  Outputs=3
  From1 : From  Commented=on  GotoTag=e  TagVisibility=global
      settings: CloseFcn=tagdialog Close
  From4 : From  Commented=on  GotoTag=io  TagVisibility=global
      settings: CloseFcn=tagdialog Close
  Mux2 : Mux  Inputs=2
  PQ_B1 : Scope  Commented=on
  "P_Q(kW, kvar)1" : Display  Commented=on
      settings: Format=bank  Decimation=2000
  Positive-Sequence Active & Reactive Power1 : Subsystem  Commented=on  AncestorBlock=|  DialogController=POWERSYS.PowerSysDialog  mask(Discrete 3-phase Positive-Sequence Active & Reactive Power){Freq=60, Par_Vinit=[0 0], Par_Iinit=[0 0], Ts=5e-6}
      | powerlib_extras/Discrete
      | Measurements/Discrete 3-phase 
      | Positive-Sequence 
      | Active & Reactive Power
      mask prompts: Freq "Fundamental frequency (Hz):"; Par_Vinit "Voltage initial input: [ Mag  Phase(degrees) ]"; Par_Iinit "Current initial input: [ Mag  Phase(degrees) ]"; Ts "Sample time:"
      mask help:
      | Measure the three-phase active power P and reactive power Q associated with a periodic set of three-phase voltages and currents which may contain harmonics. P and Q are calculated by evaluating the fundamental values (positive-sequence) of the input voltages and currents with a running window over one cycle of the fundamental frequency.
      |
      | Current flowing into an RL circuit will produce  positive active and reactive powers.
      |
      | Vabc input: Three-phase instantaneous voltage (V)
      | Iabc input: Three-phase instantaneous current (A)
      |
      | Output 1: Vector [Mag_V(V) Mag_I(A)] of the fundamental values of the voltage & current (peak values of the positive-sequence)
      | Output 2: 3-phase PQ measurement vector [P(W) Q (var)] evaluated at the fundamental frequency.
      |
      | For the first cycle of simulation, the outputs are held constant using the values specified by the parameters "Initial input".
      mask init:
      | power_initmask();
      mask Help: This block is part of a subset of blocks in the Extras library that does not have documentation associated with it, other than the block mask description.
      mask Display: disp('')
  RMS_VI2 : Scope  Commented=on
  RMS_V_I1 : Display  Commented=on
      settings: Format=bank  Decimation=2000
  Scope1 : Scope  Commented=on  NumInputPorts=2
  Scope2 : Scope
  Scope6 : Scope  NumInputPorts=2
  Terminator{1,4..6} (4 alike) : Terminator
  Terminator2 : Terminator  Commented=on
  Terminator3 : Terminator  Commented=on
  V/F : Subsystem
  wires:
  [Udc] -> V/F/4(Udc)
  Demux3/2 -> Terminator1/1
  Demux4/3 -> Terminator6/1
  [i] -> V/F/3(i)
  Demux4/2 -> Terminator5/1
  Demux4/1 -> Mux2/2
  Demux3/3 -> Terminator4/1
  From4/1 -> Scope1/2, Positive-Sequence Active & Reactive Power1/2(Iabc)
  Mux2/1 -> Scope2/1
  Demux3/1 -> Mux2/1
  Positive-Sequence Active & Reactive Power1/2(P_Q(kW)) -> PQ_B1/1, "P_Q(kW, kvar)1"/1
  Positive-Sequence Active & Reactive Power1/4(PF) -> Terminator3/1
  Positive-Sequence Active & Reactive Power1/3(Phase_V_I) -> Terminator2/1
  Positive-Sequence Active & Reactive Power1/1(RMS_V_I) -> RMS_V_I1/1, RMS_VI2/1
  From1/1 -> Scope1/1, Positive-Sequence Active & Reactive Power1/1(Vabc)
  [e] -> Scope6/1, Demux3/1, V/F/1(e)
  [io] -> Scope6/2, Demux4/1, V/F/2(io)

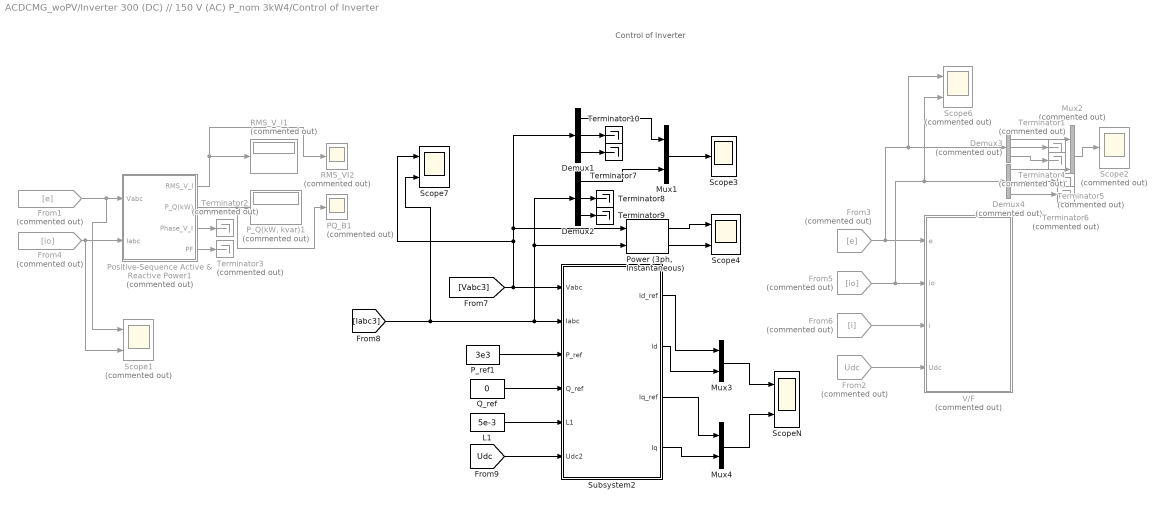
== system ACDCMG_woPV/Inverter 300 (DC) // 150 V (AC) P_nom 3kW4/Control of Inverter ==
  note: Control of Inverter
  Demux1 : Demux  Outputs=3
  Demux2 : Demux  Outputs=3
  Demux3 : Demux  Commented=on  Outputs=3
  Demux4 : Demux  Commented=on  Outputs=3
  From1 : From  Commented=on  GotoTag=e  TagVisibility=global
      settings: CloseFcn=tagdialog Close
  From2 : From  Commented=on  GotoTag=Udc  TagVisibility=global
  From3 : From  Commented=on  GotoTag=e  TagVisibility=global
  From4 : From  Commented=on  GotoTag=io  TagVisibility=global
      settings: CloseFcn=tagdialog Close
  From5 : From  Commented=on  GotoTag=io  TagVisibility=global
  From6 : From  Commented=on  GotoTag=i  TagVisibility=global
  L1 : Constant  Value=5e-3
  Mux1 : Mux  Inputs=2
  Mux2 : Mux  Commented=on  Inputs=2
  Mux3 : Mux  Inputs=2
  Mux4 : Mux  Inputs=2
  PQ_B1 : Scope  Commented=on
  "P_Q(kW, kvar)1" : Display  Commented=on
      settings: Format=bank  Decimation=2000
  P_ref1 : Constant  Value=3e3
  Positive-Sequence Active & Reactive Power1 : Subsystem  Commented=on  AncestorBlock=|  DialogController=POWERSYS.PowerSysDialog  mask(Discrete 3-phase Positive-Sequence Active & Reactive Power){Freq=60, Par_Vinit=[0 0], Par_Iinit=[0 0], Ts=5e-6}
      | powerlib_extras/Discrete
      | Measurements/Discrete 3-phase 
      | Positive-Sequence 
      | Active & Reactive Power
      mask prompts: Freq "Fundamental frequency (Hz):"; Par_Vinit "Voltage initial input: [ Mag  Phase(degrees) ]"; Par_Iinit "Current initial input: [ Mag  Phase(degrees) ]"; Ts "Sample time:"
      mask help:
      | Measure the three-phase active power P and reactive power Q associated with a periodic set of three-phase voltages and currents which may contain harmonics. P and Q are calculated by evaluating the fundamental values (positive-sequence) of the input voltages and currents with a running window over one cycle of the fundamental frequency.
      |
      | Current flowing into an RL circuit will produce  positive active and reactive powers.
      |
      | Vabc input: Three-phase instantaneous voltage (V)
      | Iabc input: Three-phase instantaneous current (A)
      |
      | Output 1: Vector [Mag_V(V) Mag_I(A)] of the fundamental values of the voltage & current (peak values of the positive-sequence)
      | Output 2: 3-phase PQ measurement vector [P(W) Q (var)] evaluated at the fundamental frequency.
      |
      | For the first cycle of simulation, the outputs are held constant using the values specified by the parameters "Initial input".
      mask init:
      | power_initmask();
      mask Help: This block is part of a subset of blocks in the Extras library that does not have documentation associated with it, other than the block mask description.
      mask Display: disp('')
  "Power (3ph, Instantaneous)" : spsPower3phInstantaneousLib/Power (3ph, Instantaneous)
  Q_ref : Constant  Value=0
  RMS_VI2 : Scope  Commented=on
  RMS_V_I1 : Display  Commented=on
      settings: Format=bank  Decimation=2000
  Scope1 : Scope  Commented=on  NumInputPorts=2
  Scope2 : Scope  Commented=on
  Scope3 : Scope
  Scope4 : Scope  NumInputPorts=2
  Scope6 : Scope  Commented=on  NumInputPorts=2
  Scope7 : Scope  NumInputPorts=2
  ScopeN : Scope  NumInputPorts=2
  Subsystem2 : Subsystem  mask{Kp=21, Ki=101, Kd=0}
      mask prompts: Kp "Proportional gain (Kp):"; Ki "Integral gain (Ki):"; Kd "Derivative gain (Kd):"
  Terminator{1..6} (6 alike) : Terminator  Commented=on
  Terminator{7..10} (4 alike) : Terminator
  V/F : Subsystem  Commented=on
  wires:
  From2/1 -> V/F/4(Udc)
  Demux3/2 -> Terminator1/1
  Demux4/3 -> Terminator6/1
  From6/1 -> V/F/3(i)
  Demux4/2 -> Terminator5/1
  Demux4/1 -> Mux2/2
  Demux3/3 -> Terminator4/1
  From4/1 -> Scope1/2, Positive-Sequence Active & Reactive Power1/2(Iabc)
  Mux2/1 -> Scope2/1
  Demux3/1 -> Mux2/1
  Positive-Sequence Active & Reactive Power1/2(P_Q(kW)) -> PQ_B1/1, "P_Q(kW, kvar)1"/1
  Positive-Sequence Active & Reactive Power1/4(PF) -> Terminator3/1
  Positive-Sequence Active & Reactive Power1/3(Phase_V_I) -> Terminator2/1
  Positive-Sequence Active & Reactive Power1/1(RMS_V_I) -> RMS_V_I1/1, RMS_VI2/1
  From1/1 -> Scope1/1, Positive-Sequence Active & Reactive Power1/1(Vabc)
  From3/1 -> Scope6/1, Demux3/1, V/F/1(e)
  From5/1 -> Scope6/2, Demux4/1, V/F/2(io)
  Q_ref/1 -> Subsystem2/4(Q_ref)
  [Vabc3] -> Subsystem2/1(Vabc), Scope7/1, Demux1/1, "Power (3ph, Instantaneous)"/1
  Demux2/3 -> Terminator9/1
  Demux1/2 -> Terminator10/1
  [Udc] -> Subsystem2/6(Udc2)
  P_ref1/1 -> Subsystem2/3(P_ref)
  Demux2/2 -> Terminator8/1
  "Power (3ph, Instantaneous)"/2 -> Scope4/2
  "Power (3ph, Instantaneous)"/1 -> Scope4/1
  Subsystem2/3(Iq_ref) -> Mux4/1
  Subsystem2/2(Id) -> Mux3/2
  Demux2/1 -> Mux1/2
  Mux1/1 -> Scope3/1
  L1/1 -> Subsystem2/5(L1)
  Mux3/1 -> ScopeN/1
  Subsystem2/4(Iq) -> Mux4/2
  [Iabc3] -> Scope7/2, Demux2/1, "Power (3ph, Instantaneous)"/2, Subsystem2/2(Iabc)
  Subsystem2/1(Id_ref) -> Mux3/1
  Mux4/1 -> ScopeN/2
  Demux1/3 -> Terminator7/1
  Demux1/1 -> Mux1/1

== system ACDCMG_woPV/M1/Power Factor Block1 ==
  Vabc : Inport
  Iabc : Inport  Port=2
  Complex to Magnitude-Angle : ComplexToMagnitudeAngle
  Conv pu1 : Gain  Gain=sqrt (3) /Vnom_prim  SaturateOnIntegerOverflow=on  OutDataTypeStr=Inherit: Same as input  ParamDataTypeStr=Inherit: Same as input
  Gain1 : Gain  Gain=-1/1000
  Mux : Mux  Inputs=2
  Power : spsPowerLib/Power  Freq=Freq  Vinit=Vinit  Iinit=Iinit  Ts=Ts
      settings: SourceProductBaseCode=PS
  Real-Imag to Complex : RealImagToComplex
  Terminator : Terminator
  cos(theta) : Trigonometry  Operator=cos
  to Kw : Gain  Gain=-1/1000
  "Vabc y Vabc " : Outport  VectorParamsAs1DForOutWhenUnconnected=off
  "Iabc y Iabc " : Outport  Port=2  VectorParamsAs1DForOutWhenUnconnected=off
  Outport : Outport  Port=3
  tag scope: P_abc_Bus9=global, Q_abc_Bus9=global, Vabc_LL_pu_Bus9=global
  wires:
  Power/1 -> Gain1/1, Real-Imag to Complex/1
  Power/2 -> Real-Imag to Complex/2, to Kw/1
  Complex to Magnitude-Angle/2 -> cos(theta)/1
  Real-Imag to Complex/1 -> Complex to Magnitude-Angle/1
  cos(theta)/1 -> Outport/1
  Complex to Magnitude-Angle/1 -> Terminator/1
  Iabc/1 -> "Iabc y Iabc "/1, Power/2
  Mux/1 -> "Vabc y Vabc "/1
  Vabc/1 -> Power/1, Conv pu1/1, Mux/1, Mux/2
  Conv pu1/1 -> [Vabc_LL_pu_Bus9]
  to Kw/1 -> [Q_abc_Bus9]
  Gain1/1 -> [P_abc_Bus9]

== system ACDCMG_woPV/M2/Power Factor Block1 ==
  Vabc : Inport
  Iabc : Inport  Port=2
  Complex to Magnitude-Angle : ComplexToMagnitudeAngle  Commented=on
  Conv pu1 : Gain  Gain=sqrt (3) /Vnom_sec  SaturateOnIntegerOverflow=on  OutDataTypeStr=Inherit: Same as input  ParamDataTypeStr=Inherit: Same as input
  Current1 : Goto  Commented=on  GotoTag=P_abc_Bus1  TagVisibility=global
  Current2 : Goto  Commented=on  GotoTag=Q_abc_Bus1  TagVisibility=global
  Gain1 : Gain  Commented=on  Gain=-1/1000
  Mux : Mux  Inputs=2
  Power : spsPowerLib/Power  Commented=on  Freq=Freq  Vinit=Vinit  Iinit=Iinit  Ts=Ts
      settings: SourceProductBaseCode=PS
  Real-Imag to Complex : RealImagToComplex  Commented=on
  Terminator : Terminator  Commented=on
  cos(theta) : Trigonometry  Commented=on  Operator=cos
  to Kw : Gain  Commented=on  Gain=-1/1000
  "Vabc y Vabc " : Outport  VectorParamsAs1DForOutWhenUnconnected=off
  "Iabc y Iabc " : Outport  Port=2  VectorParamsAs1DForOutWhenUnconnected=off
  tag scope: Vabc_LL_pu_Bus1=global
  wires:
  Power/1 -> Gain1/1, Real-Imag to Complex/1
  Power/2 -> Real-Imag to Complex/2, to Kw/1
  Complex to Magnitude-Angle/2 -> cos(theta)/1
  Real-Imag to Complex/1 -> Complex to Magnitude-Angle/1
  Complex to Magnitude-Angle/1 -> Terminator/1
  Iabc/1 -> "Iabc y Iabc "/1, Power/2
  Mux/1 -> "Vabc y Vabc "/1
  Vabc/1 -> Power/1, Conv pu1/1, Mux/1, Mux/2
  Conv pu1/1 -> [Vabc_LL_pu_Bus1]
  to Kw/1 -> Current2/1
  Gain1/1 -> Current1/1

== system ACDCMG_woPV/M4/Power Factor Block1 ==
  Vabc : Inport
  Iabc : Inport  Port=2
  Complex to Magnitude-Angle : ComplexToMagnitudeAngle  Commented=on
  Conv pu2 : Gain  Gain=sqrt (3) /Vnom_prim  SaturateOnIntegerOverflow=on  OutDataTypeStr=Inherit: Same as input  ParamDataTypeStr=Inherit: Same as input
  Current3 : Goto  Commented=on  GotoTag=P_abc_Bus6  TagVisibility=global
  Current4 : Goto  Commented=on  GotoTag=Q_abc_Bus6  TagVisibility=global
  Mux : Mux  Inputs=2
  Power : spsPowerLib/Power  Freq=Freq  Vinit=Vinit  Iinit=Iinit  Ts=Ts
      settings: SourceProductBaseCode=PS
  Real-Imag to Complex : RealImagToComplex  Commented=on
  cos(theta) : Trigonometry  Commented=on  Operator=cos
  to Kw : Gain  Commented=on  Gain=1/1000
  to Kw1 : Gain  Commented=on  Gain=1/1000
  "Vabc y Vabc " : Outport  VectorParamsAs1DForOutWhenUnconnected=off
  "Iabc y Iabc " : Outport  Port=2  VectorParamsAs1DForOutWhenUnconnected=off
  tag scope: Vabc_LL_pu_Bus6=global
  wires:
  Complex to Magnitude-Angle/2 -> cos(theta)/1
  Real-Imag to Complex/1 -> Complex to Magnitude-Angle/1
  Iabc/1 -> "Iabc y Iabc "/1, Power/2
  Mux/1 -> "Vabc y Vabc "/1
  Vabc/1 -> Power/1, Conv pu2/1, Mux/1, Mux/2
  Conv pu2/1 -> [Vabc_LL_pu_Bus6]
  Power/2 -> Real-Imag to Complex/2, to Kw/1
  Power/1 -> to Kw1/1, Real-Imag to Complex/1
  to Kw/1 -> Current4/1
  to Kw1/1 -> Current3/1

== system ACDCMG_woPV/Resource1/Irradiance Temp Demand Max ==
  Demux : Demux  Tag=STV Demux  Outputs=2
      settings: DisplayOption=none
  FromWs : FromWorkspace  Tag=STV FromWs  VariableName=tuvar
      SigBuilderData=|
      | common.afterFinalStr = 'Extrapolate'
      | common.sampleTime = '0'
      | dataSet(1).timeRange = [0 2]
      | dataSet(1).name = 'Constant Irradiance'
      | dataSet(2).timeRange = [0 2]
      | dataSet(2).name = 'Step Irradiance'
      | dataSet(3).timeRange = [0 3]
      | dataSet(3).name = 'Ramp-up/down Irradiance'
      | sbobj.Groups(1).Name = 'Constant Irradiance'
      | sbobj.Groups(1).Signals(1).Name = 'Ir'
      | sbobj.Groups(1).Signals(1).XData = [0 2]
      | sbobj.Groups(1).Signals(1).YData = [1000 1000]
      | sbobj.Groups(1).Signals(2).Name = 'Temp'
      | sbobj.Groups(1).Signals(2).XData = [0 1 1 2]
      | sbobj.Groups(1).Signals(2).YData = [0 0 1 1]
      | sbobj.Groups(1).TimeRange = [0 2]
      | sbobj.Groups(2).Name = 'Step Irradiance'
      | sbobj.Groups(2).Signals(1).Name = 'Ir'
      | sbobj.Groups(2).Signals(1).XData = [0 0.252 0.252 2]
      | sbobj.Groups(2).Signals(1).YData = [600 600 1000 1000]
      | sbobj.Groups(2).Signals(2).Name = 'Temp'
      | sbobj.Groups(2).Signals(2).XData = [0 1 1 2]
      | sbobj.Groups(2).Signals(2).YData = [0 0 1 1]
      | sbobj.Groups(2).TimeRange = [0 2]
      | sbobj.Groups(3).Name = 'Ramp-up/down Irradiance'
      | sbobj.Groups(3).Signals(1).Name = 'Ir'
      | sbobj.Groups(3).Signals(1).XData = [0 0.785 1.7 2.28 3]
      | sbobj.Groups(3).Signals(1).YData = [1000 999.538235294 999 999.446153846 1000]
      | sbobj.Groups(3).Signals(2).Name = 'Temp'
      | sbobj.Groups(3).Signals(2).XData = [0 2 2.1 3]
      | sbobj.Groups(3).Signals(2).YData = [25 25 25 25]
      | sbobj.Groups(3).TimeRange = [0 3]
  Ir : Outport  Tag=STV Outport  VectorParamsAs1DForOutWhenUnconnected=off
  Temp : Outport  Tag=STV Outport  Port=2  VectorParamsAs1DForOutWhenUnconnected=off
  wires:
  Demux/1 -> Ir/1
  FromWs/1 -> Demux/1
  Demux/2 -> Temp/1

== system ACDCMG_woPV/Smart Meter: Grid /Power Factor Block1 ==
  Vabc : Inport
  Iabc : Inport  Port=2
  Complex to Magnitude-Angle : ComplexToMagnitudeAngle  Commented=on
  Conv pu2 : Gain  Gain=sqrt (3) /Vnom_prim  SaturateOnIntegerOverflow=on  OutDataTypeStr=Inherit: Same as input  ParamDataTypeStr=Inherit: Same as input
  Current3 : Goto  Commented=on  GotoTag=P_abc_Bus3  TagVisibility=global
  Current4 : Goto  Commented=on  GotoTag=Q_abc_Bus3  TagVisibility=global
  Gain : Gain  Commented=on  Gain=-1/1000
  Gain1 : Gain  Commented=on  Gain=-1/1000
  Mux : Mux  Inputs=2
  Power : spsPowerLib/Power  Commented=on  Freq=Freq  Vinit=Vinit  Iinit=Iinit  Ts=Ts
      settings: SourceProductBaseCode=PS
  Real-Imag to Complex : RealImagToComplex  Commented=on
  Terminator : Terminator  Commented=on
  cos(theta) : Trigonometry  Commented=on  Operator=cos
  "Vabc y Vabc " : Outport  VectorParamsAs1DForOutWhenUnconnected=off
  "Iabc y Iabc " : Outport  Port=2  VectorParamsAs1DForOutWhenUnconnected=off
  tag scope: Vabc_LL_pu_Bus3=global
  wires:
  Complex to Magnitude-Angle/2 -> cos(theta)/1
  Real-Imag to Complex/1 -> Complex to Magnitude-Angle/1
  cos(theta)/1 -> ?
  Complex to Magnitude-Angle/1 -> Terminator/1
  Iabc/1 -> "Iabc y Iabc "/1, Power/2
  Mux/1 -> "Vabc y Vabc "/1
  Vabc/1 -> Power/1, Conv pu2/1, Mux/1, Mux/2
  Conv pu2/1 -> [Vabc_LL_pu_Bus3]
  Power/1 -> Gain/1, Real-Imag to Complex/1
  Power/2 -> Real-Imag to Complex/2, Gain1/1
  Gain1/1 -> Current4/1
  Gain/1 -> Current3/1

== system ACDCMG_woPV/Smart Meter: Unbalanced Load/Power Factor Block1 ==
  Vabc : Inport
  Iabc : Inport  Port=2
  Complex to Magnitude-Angle : ComplexToMagnitudeAngle  Commented=on
  Power : spsPowerLib/Power  Commented=on  Freq=Freq  Vinit=Vinit  Iinit=Iinit  Ts=Ts
      settings: SourceProductBaseCode=PS
  Real-Imag to Complex : RealImagToComplex  Commented=on
  Terminator : Terminator  Commented=on
  cos(theta) : Trigonometry  Commented=on  Operator=cos
  Vabc y Vabc : Outport  VectorParamsAs1DForOutWhenUnconnected=off
  "Iabc y Iabc " : Outport  Port=2  VectorParamsAs1DForOutWhenUnconnected=off
  wires:
  Power/1 -> Real-Imag to Complex/1
  Power/2 -> Real-Imag to Complex/2
  Complex to Magnitude-Angle/2 -> cos(theta)/1
  Real-Imag to Complex/1 -> Complex to Magnitude-Angle/1
  cos(theta)/1 -> ?
  Complex to Magnitude-Angle/1 -> Terminator/1
  Iabc/1 -> "Iabc y Iabc "/1, Power/2
  Vabc/1 -> Vabc y Vabc/1, Power/1

== system ACDCMG_woPV/Boost -buck Bi-directional converter 1 0.65 kW/+ve reference For Buck --> -ve reference For Boost <--/PID Orig Boost ==
  error : Inport
  Integrator2 : Integrator  LimitOutput=on  UpperSaturationLimit=0.9  LowerSaturationLimit=0
  Ki2 : Gain  Gain=3
  Kp2 : Gain  Gain=0.02
  Sum4 : Sum  Inputs=|++
  Out1 : Outport  VectorParamsAs1DForOutWhenUnconnected=off
  wires:
  error/1 -> Kp2/1, Ki2/1
  Kp2/1 -> Sum4/1
  Sum4/1 -> Out1/1
  Ki2/1 -> Integrator2/1
  Integrator2/1 -> Sum4/2

== system ACDCMG_woPV/Boost -buck Bi-directional converter 1 0.65 kW/+ve reference For Buck --> -ve reference For Boost <--/PID Orig Buck ==
  error : Inport
  Integrator3 : Integrator  LimitOutput=on  UpperSaturationLimit=0.9  LowerSaturationLimit=0
  Ki3 : Gain  Gain=110
  Kp3 : Gain  Gain=0.2
  Sum1 : Sum  Inputs=|++
  Out1 : Outport  VectorParamsAs1DForOutWhenUnconnected=off
  wires:
  Integrator3/1 -> Sum1/2
  Ki3/1 -> Integrator3/1
  Kp3/1 -> Sum1/1
  Sum1/1 -> Out1/1
  error/1 -> Kp3/1, Ki3/1

== system ACDCMG_woPV/Boost -buck Bi-directional converter 1 0.65 kW/Primary Control/PID Orig Boost ==
  error : Inport
  Delay : Delay  DelayLength=1  InitialCondition=0  SampleTime=Ts
  Integrator : Integrator  InitialCondition=0.1  LimitOutput=on  UpperSaturationLimit=0.9  LowerSaturationLimit=0.1
  Ki : Gain  Gain=0.001
  Kp : Gain  Gain=0.000005
  Kp1 : Gain  Gain=60
  Sum1 : Sum  Inputs=|++
  Out1 : Outport  VectorParamsAs1DForOutWhenUnconnected=off
  wires:
  Integrator/1 -> Sum1/2
  Sum1/1 -> Out1/1
  Ki/1 -> Integrator/1
  Kp/1 -> Sum1/1
  error/1 -> Delay/1
  Delay/1 -> Kp1/1
  Kp1/1 -> Kp/1, Ki/1

== system ACDCMG_woPV/Boost -buck Bi-directional converter DC //DC 1 0.65 kW Switching Model/+ve reference For Buck --> -ve reference For Boost <--/PID Orig Boost ==
  error : Inport
  Integrator2 : Integrator  LimitOutput=on  UpperSaturationLimit=0.9  LowerSaturationLimit=0
  Ki2 : Gain  Gain=3
  Kp2 : Gain  Gain=0.02
  Sum4 : Sum  Inputs=|++
  Out1 : Outport  VectorParamsAs1DForOutWhenUnconnected=off
  wires:
  error/1 -> Kp2/1, Ki2/1
  Kp2/1 -> Sum4/1
  Sum4/1 -> Out1/1
  Ki2/1 -> Integrator2/1
  Integrator2/1 -> Sum4/2

== system ACDCMG_woPV/Boost -buck Bi-directional converter DC //DC 1 0.65 kW Switching Model/+ve reference For Buck --> -ve reference For Boost <--/PID Orig Buck ==
  error : Inport
  Integrator3 : Integrator  LimitOutput=on  UpperSaturationLimit=0.9  LowerSaturationLimit=0
  Ki3 : Gain  Gain=110
  Kp3 : Gain  Gain=0.2
  Sum1 : Sum  Inputs=|++
  Out1 : Outport  VectorParamsAs1DForOutWhenUnconnected=off
  wires:
  Integrator3/1 -> Sum1/2
  Ki3/1 -> Integrator3/1
  Kp3/1 -> Sum1/1
  Sum1/1 -> Out1/1
  error/1 -> Kp3/1, Ki3/1
